simulink model "lab"  (R2018b)
settings: Solver=FixedStepAuto  StartTime=0.0  StopTime=10.0  FixedStep=0.01  RelTol=1e-3
undefined symbols (not defined in the file or in its folder): G, s
settings Model: Creator=Oguz  LastModifiedBy=Oguz

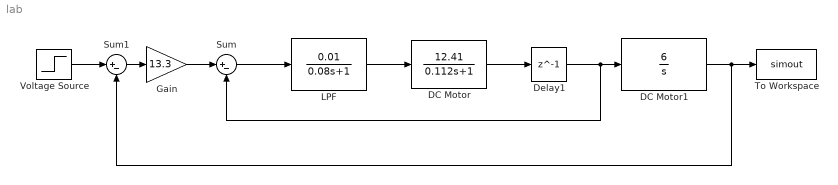
== system lab ==
  DC Motor : TransferFcn  Numerator=[12.41]  Denominator=[0.112 1]  ContinuousStateAttributes=G(s)
  DC Motor1 : TransferFcn  Numerator=[6]  Denominator=[1 0]
  Delay1 : Delay  DelayLength=1
  Gain : Gain  Gain=13.3
  "LPF " : TransferFcn  Numerator=[0.01]  Denominator=[0.08 1]
  Sum : Sum  Inputs=|+-
  Sum1 : Sum  Inputs=|+-
  To Workspace : ToWorkspace  VariableName=simout  SaveFormat=Timeseries  SampleTime=-1
  "Voltage Source " : Step  Time=0  After=90  SampleTime=0
  wires:
  Gain/1 -> Sum/1
  "LPF "/1 -> DC Motor/1
  Sum/1 -> "LPF "/1
  "Voltage Source "/1 -> Sum1/1
  Sum1/1 -> Gain/1
  DC Motor/1 -> Delay1/1
  DC Motor1/1 -> Sum1/2, To Workspace/1
  Delay1/1 -> DC Motor1/1, Sum/2
